simulink model "mod_observer_unit_test"  (R2015a)
settings: Solver=ode3  StartTime=0.0  StopTime=750  FixedStep=0.01  RelTol=1e-3
libraries: simulink x3
settings Model: Creator=MCLab  LastModifiedBy=MCLab

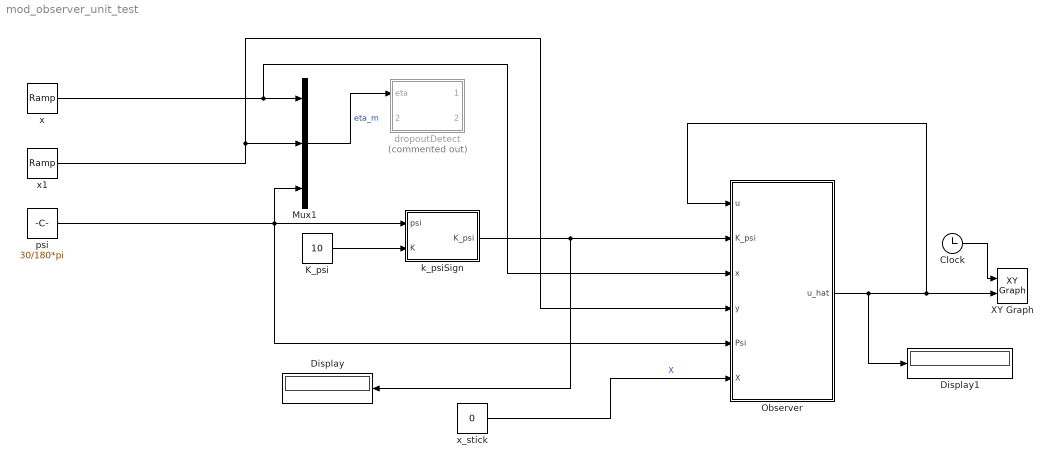
== system mod_observer_unit_test ==
  Clock : Clock
  Display : Display
  Display1 : Display
  K_psi : Constant  Value=10
  Mux1 : Mux  Inputs=3
  Observer : Subsystem
  XY Graph : simulink/Sinks/XY Graph  xmin=0  xmax=100  ymin=-0.15  ymax=.15  st=-1
  dropoutDetect : MATLAB Function  Commented=on  TreatAsAtomicUnit=on
  k_psiSign : MATLAB Function  TreatAsAtomicUnit=on
  psi : Constant  Value=30/180*pi
  x : simulink/Sources/Ramp  slope=0.1  start=0.2  X0=0
  x1 : simulink/Sources/Ramp  slope=0  start=0.2  X0=0
  "x_stick " : Constant  Value=0
  wires:
  x/1 -> Mux1/1, Observer/3(x)
  x1/1 -> Observer/4("y "), Mux1/2
  psi/1 -> Observer/5(Psi), Mux1/3, k_psiSign/1(psi)
  "x_stick "/1 -> Observer/6(X)  "X"
  k_psiSign/1(K_psi) -> Display/1, Observer/2(K_psi)
  K_psi/1 -> k_psiSign/2(K)
  Mux1/1 -> dropoutDetect/1(eta)  "eta_m"
  Clock/1 -> XY Graph/1
  Observer/1(u_hat) -> Display1/1, Observer/1(u), XY Graph/2

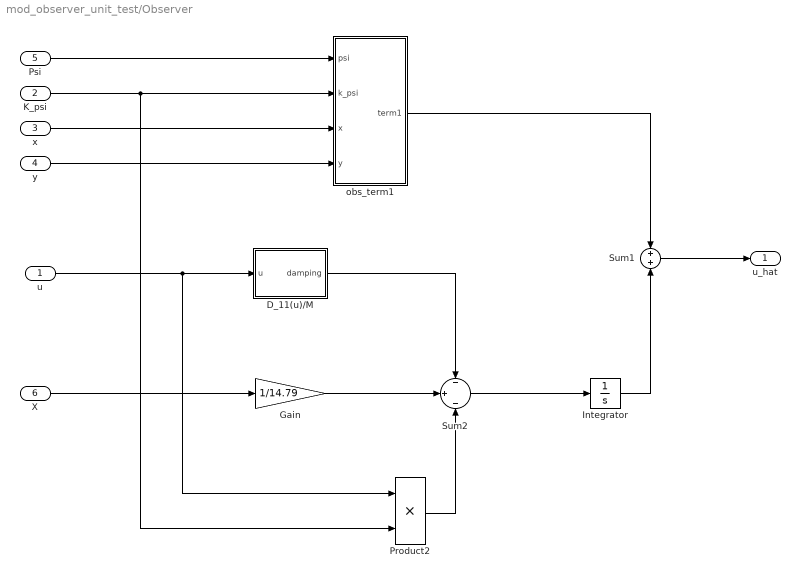
== system mod_observer_unit_test/Observer ==
  u : Inport
  K_psi : Inport  Port=2
  x : Inport  Port=3
  "y " : Inport  Port=4
  Psi : Inport  Port=5
  X : Inport  Port=6
  D_11(u)/M : MATLAB Function  TreatAsAtomicUnit=on
  Gain : Gain  Gain=1/14.79
  Integrator : Integrator
  Product2 : Product
  Sum1 : Sum  Inputs=+|+
  Sum2 : Sum  Inputs=-|+|-
  obs_term1 : MATLAB Function  TreatAsAtomicUnit=on
  u_hat : Outport
  wires:
  x/1 -> obs_term1/3(x)
  Sum1/1 -> u_hat/1
  Sum2/1 -> Integrator/1
  Integrator/1 -> Sum1/2
  "y "/1 -> obs_term1/4(y)
  u/1 -> Product2/1, D_11(u)/M/1(u)
  D_11(u)/M/1(damping) -> Sum2/1
  X/1 -> Gain/1
  Gain/1 -> Sum2/2
  Psi/1 -> obs_term1/1(psi)
  K_psi/1 -> obs_term1/2(k_psi), Product2/2
  Product2/1 -> Sum2/3
  obs_term1/1(term1) -> Sum1/1

== matlab function mod_observer_unit_test/k_psiSign ==
  data: psi input; K input; K_psi output
function K_psi = fcn(psi,K)

K_psi=K;
%K_psi=K*sign(cos(psi)+sin(psi));



end

== matlab function mod_observer_unit_test/Observer/D_11(u)//M ==
  data: u input; damping output
function damping = fcn(u)
%#codegen
%y = u;
damping=(0.6555-0.3545*abs(u)+3.787*u^2)*u/14.79;

end

== matlab function mod_observer_unit_test/Observer/obs_term1 ==
  data: psi input; term1 output; k_psi input; x input; y input
function term1 = fcn(psi,k_psi,x,y)

term1=k_psi*(x*cos(psi)+y*sin(psi));

end

== matlab function mod_observer_unit_test/dropoutDetect ==
  data: eta input; dropout output; etaPrev input; etaOut output
function [dropout,etaOut]= fcn(eta,etaPrev)




end
